simulink model "I_Erweiterung"  (R2019a)
settings: Solver=VariableStepAuto  StartTime=0.0  StopTime=10.0  RelTol=1e-3
values from neighbouring files (symbols this model uses):
  A = [0 1 0 0;m*g*l(M+m)/d 0 0 m*l*b/d;0 0 0 1;-g*m^2*l^2/d 0 0 -b*(I+m*l^2)/d]    [inv_pend.m]
  B = [0;-m*l/d;0;(I+m*l^2)/d]    [inv_pend.m]
  C = [0 0 1 0;1 0 0 0]    [inv_pend.m]
  K1 = KI(:,1:end-size(Cn,1))    [inv_pend.m]
  K2 = KI(:,end-size(Cn,1)+1:end)    [inv_pend.m]
settings Model: Creator=Naveen  LastModifiedBy=Naveen

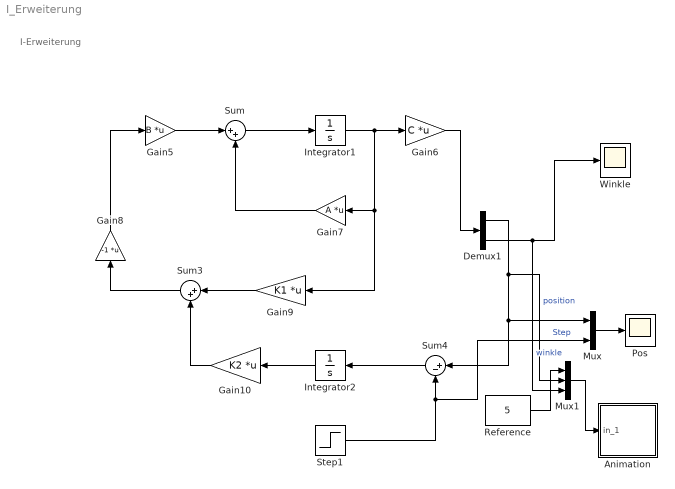
== system I_Erweiterung ==
  note: I-Erweiterung
  Animation : Subsystem  mask(Pendulum plot){RefBlock=Reference}
      mask prompts: RefBlock "DC reference signal block name:"
      mask help: Pendulum plot
      mask Help: Pendulum animation function using Handle graphics.
      mask Display: plot([-10 10],[0 0],[-2 -2 2 2],[0 1 1 0],[0 3],[1 5])
  Demux1 : Demux  Outputs=2
  Gain10 : Gain  Gain=K2  Multiplication=Matrix(K*u)
  Gain5 : Gain  Gain=B  Multiplication=Matrix(K*u)
  Gain6 : Gain  Gain=C  Multiplication=Matrix(K*u)
  Gain7 : Gain  Gain=A  Multiplication=Matrix(K*u)
  Gain8 : Gain  Gain=-1  Multiplication=Matrix(K*u)
  Gain9 : Gain  Gain=K1  Multiplication=Matrix(K*u)
  Integrator1 : Integrator
  Integrator2 : Integrator
  Mux : Mux  Inputs=2
  Mux1 : Mux  Inputs=3
  Pos : Scope
  Reference : Constant  Value=5
  Step1 : Step  Time=0  After=5  SampleTime=0
  Sum : Sum  Inputs=|++
  Sum3 : Sum  Inputs=|++
  Sum4 : Sum  Inputs=|+-
  Winkle : Scope
  wires:
  Sum3/1 -> Gain8/1
  Gain10/1 -> Sum3/2
  Gain9/1 -> Sum3/1
  Sum/1 -> Integrator1/1
  Gain5/1 -> Sum/1
  Integrator2/1 -> Gain10/1
  Gain8/1 -> Gain5/1
  Integrator1/1 -> Gain9/1, Gain7/1, Gain6/1
  Step1/1 -> Mux/2, Sum4/2  "Step"
  Mux/1 -> Pos/1
  Gain7/1 -> Sum/2
  Gain6/1 -> Demux1/1
  Sum4/1 -> Integrator2/1
  Reference/1 -> Mux1/1
  Demux1/2 -> Mux1/3, Winkle/1  "winkle"
  Mux1/1 -> Animation/1(in_1)
  Demux1/1 -> Mux1/2, Mux/1, Sum4/1  "position"

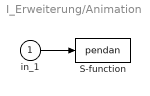
== system I_Erweiterung/Animation ==
  in_1 : Inport
  S-function : S-Function  FunctionName=pendan  Parameters=RefBlock  SFunctionDeploymentMode=off  EnableBusSupport=off
      settings: DeleteFcn=pendan([],[],[],'DeleteBlock');
  wires:
  in_1/1 -> S-function/1
